simulink model "Cascade_control_simulink"  (R2023a)
settings: Solver=VariableStepAuto  StartTime=0.0  StopTime=100  RelTol=1e-3
settings Model: Creator=owner  LastModifiedBy=owner

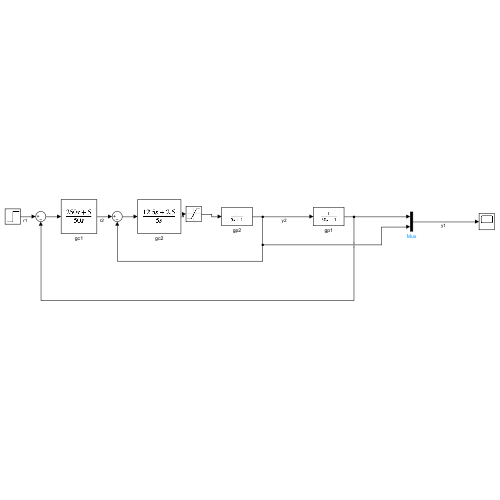
[thumbnail: Simulink's stored preview of the top-level diagram]
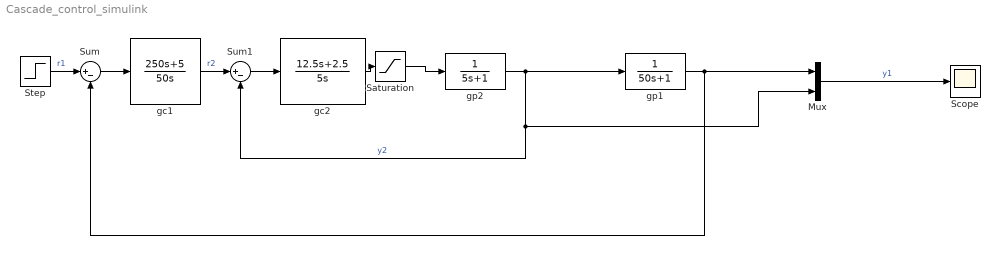
== system Cascade_control_simulink ==
  Mux : Mux  Inputs=2
  Saturation : Saturate  UpperLimit=3  LowerLimit=-3
  Scope : Scope
  Step : Step  SampleTime=0
  Sum : Sum  Inputs=|+-
  Sum1 : Sum  Inputs=|+-
  gc1 : TransferFcn  Numerator=[250 5]  Denominator=[50 0]
  gc2 : TransferFcn  Numerator=[12.5 2.5]  Denominator=[5 0]
  gp1 : TransferFcn  Denominator=[50 1]
  gp2 : TransferFcn  Denominator=[5 1]
  wires:
  Sum/1 -> gc1/1
  gc1/1 -> Sum1/1  "r2"
  Step/1 -> Sum/1  "r1"
  gc2/1 -> Saturation/1
  Sum1/1 -> gc2/1
  gp2/1 -> Sum1/2, Mux/2, gp1/1  "y2"
  gp1/1 -> Sum/2, Mux/1
  Saturation/1 -> gp2/1
  Mux/1 -> Scope/1  "y1"
